simulink model "TrackShift_F1_HEV"  (R2025a)
settings: Solver=FixedStepDiscrete  StartTime=0.0  StopTime=90  FixedStep=0.25  RelTol=1e-3
model workspace (MAT data in the model file):
  TS_BRAKE = [0 0.25 0.5 0.75 1 1.25 1.5 1.75 2 2.25 2.5 2.75 ... (722 elements, 361x2)]
  TS_ENGINE_CAPACITY_L = 1.6
  TS_GAP_S = [0 0.25 0.5 0.75 1 1.25 1.5 1.75 2 2.25 2.5 2.75 ... (722 elements, 361x2)]
  TS_GRADIENT_RAD = [0 0.25 0.5 0.75 1 1.25 1.5 1.75 2 2.25 2.5 2.75 ... (722 elements, 361x2)]
  TS_HANDOVER_SOURCE = 'handover.rar / handover/export/models (production logistic models)'
  TS_SAMPLE_TIME_S = 0.25
  TS_SPEED_KPH = [0 0.25 0.5 0.75 1 1.25 1.5 1.75 2 2.25 2.5 2.75 ... (722 elements, 361x2)]
  TS_THROTTLE = [0 0.25 0.5 0.75 1 1.25 1.5 1.75 2 2.25 2.5 2.75 ... (722 elements, 361x2)]
  TS_TRACK_POS_M = [0 0.25 0.5 0.75 1 1.25 1.5 1.75 2 2.25 2.5 2.75 ... (722 elements, 361x2)]
(part 1 of 2)
settings Model: Creator=Navya  LastModifiedBy=Navya

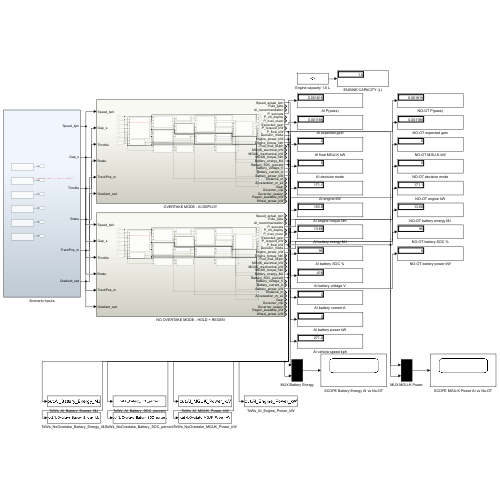
[thumbnail: Simulink's stored preview of the top-level diagram]
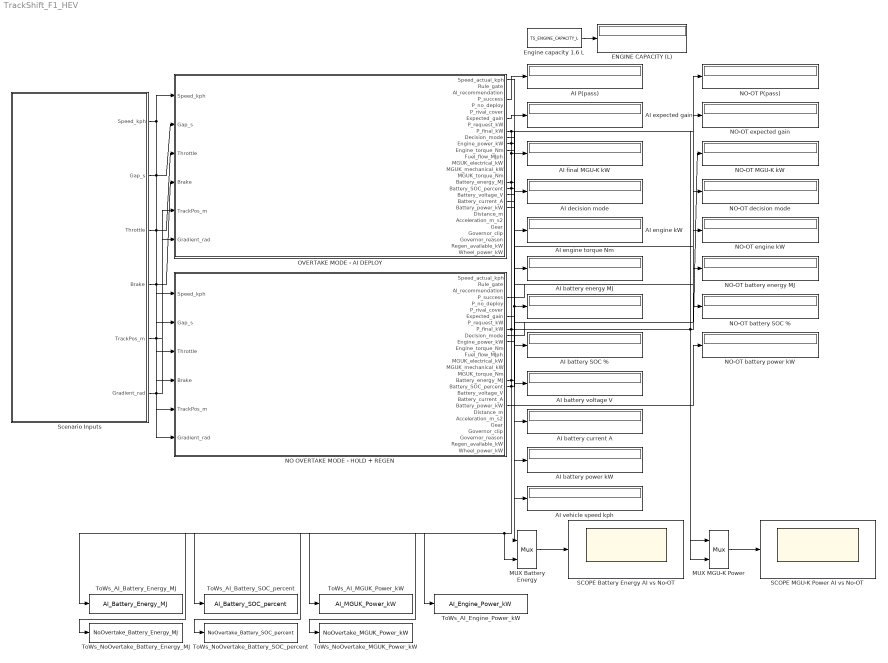
== system TrackShift_F1_HEV ==
  AI P(pass) : Display
  AI battery SOC % : Display
  AI battery current A : Display
  AI battery energy MJ : Display
  AI battery power kW : Display
  AI battery voltage V : Display
  AI decision mode : Display
  AI engine kW : Display
  AI engine torque Nm : Display
  AI expected gain : Display
  AI final MGU-K kW : Display
  AI vehicle speed kph : Display
  ENGINE CAPACITY (L) : Display
  Engine capacity 1.6 L : Constant  Value=TS_ENGINE_CAPACITY_L
  MUX Battery Energy : Mux  Inputs=2
  MUX MGU-K Power : Mux  Inputs=2
  NO OVERTAKE MODE - HOLD + REGEN : Subsystem
  NO-OT MGU-K kW : Display
  NO-OT P(pass) : Display
  NO-OT battery SOC % : Display
  NO-OT battery energy MJ : Display
  NO-OT battery power kW : Display
  NO-OT decision mode : Display
  NO-OT engine kW : Display
  NO-OT expected gain : Display
  OVERTAKE MODE - AI DEPLOY : Subsystem
  SCOPE Battery Energy AI vs No-OT : Scope
      settings: ActiveDisplayYMinimum=11.25  ActiveDisplayYMaximum=13.950000000000001
  SCOPE MGU-K Power AI vs No-OT : Scope
      settings: ActiveDisplayYMinimum=-169.375  ActiveDisplayYMaximum=324.375
  Scenario Inputs : Subsystem
  ToWs_AI_Battery_Energy_MJ : ToWorkspace  VariableName=AI_Battery_Energy_MJ  SaveFormat=Structure With Time  SampleTime=-1
  ToWs_AI_Battery_SOC_percent : ToWorkspace  VariableName=AI_Battery_SOC_percent  SaveFormat=Structure With Time  SampleTime=-1
  ToWs_AI_Engine_Power_kW : ToWorkspace  VariableName=AI_Engine_Power_kW  SaveFormat=Structure With Time  SampleTime=-1
  ToWs_AI_MGUK_Power_kW : ToWorkspace  VariableName=AI_MGUK_Power_kW  SaveFormat=Structure With Time  SampleTime=-1
  ToWs_NoOvertake_Battery_Energy_MJ : ToWorkspace  VariableName=NoOvertake_Battery_Energy_MJ  SaveFormat=Structure With Time  SampleTime=-1
  ToWs_NoOvertake_Battery_SOC_percent : ToWorkspace  VariableName=NoOvertake_Battery_SOC_percent  SaveFormat=Structure With Time  SampleTime=-1
  ToWs_NoOvertake_MGUK_Power_kW : ToWorkspace  VariableName=NoOvertake_MGUK_Power_kW  SaveFormat=Structure With Time  SampleTime=-1
  wires:
  Scenario Inputs/1(Speed_kph) -> OVERTAKE MODE - AI DEPLOY/1(Speed_kph), NO OVERTAKE MODE - HOLD + REGEN/1(Speed_kph)
  Scenario Inputs/2(Gap_s) -> OVERTAKE MODE - AI DEPLOY/2(Gap_s), NO OVERTAKE MODE - HOLD + REGEN/2(Gap_s)
  Scenario Inputs/3(Throttle) -> OVERTAKE MODE - AI DEPLOY/3(Throttle), NO OVERTAKE MODE - HOLD + REGEN/3(Throttle)
  Scenario Inputs/4(Brake) -> OVERTAKE MODE - AI DEPLOY/4(Brake), NO OVERTAKE MODE - HOLD + REGEN/4(Brake)
  Scenario Inputs/5(TrackPos_m) -> OVERTAKE MODE - AI DEPLOY/5(TrackPos_m), NO OVERTAKE MODE - HOLD + REGEN/5(TrackPos_m)
  Scenario Inputs/6(Gradient_rad) -> OVERTAKE MODE - AI DEPLOY/6(Gradient_rad), NO OVERTAKE MODE - HOLD + REGEN/6(Gradient_rad)
  Engine capacity 1.6 L/1 -> ENGINE CAPACITY (L)/1
  OVERTAKE MODE - AI DEPLOY/4(P_success) -> AI P(pass)/1
  OVERTAKE MODE - AI DEPLOY/7(Expected_gain) -> AI expected gain/1
  OVERTAKE MODE - AI DEPLOY/9(P_final_kW) -> AI final MGU-K kW/1, ToWs_AI_MGUK_Power_kW/1, MUX MGU-K Power/1
  OVERTAKE MODE - AI DEPLOY/10(Decision_mode) -> AI decision mode/1
  OVERTAKE MODE - AI DEPLOY/11(Engine_power_kW) -> AI engine kW/1, ToWs_AI_Engine_Power_kW/1
  OVERTAKE MODE - AI DEPLOY/12(Engine_torque_Nm) -> AI engine torque Nm/1
  OVERTAKE MODE - AI DEPLOY/17(Battery_energy_MJ) -> AI battery energy MJ/1, MUX Battery Energy/1, ToWs_AI_Battery_Energy_MJ/1
  OVERTAKE MODE - AI DEPLOY/18(Battery_SOC_percent) -> AI battery SOC %/1, ToWs_AI_Battery_SOC_percent/1
  OVERTAKE MODE - AI DEPLOY/19(Battery_voltage_V) -> AI battery voltage V/1
  OVERTAKE MODE - AI DEPLOY/20(Battery_current_A) -> AI battery current A/1
  OVERTAKE MODE - AI DEPLOY/21(Battery_power_kW) -> AI battery power kW/1
  OVERTAKE MODE - AI DEPLOY/1(Speed_actual_kph) -> AI vehicle speed kph/1
  NO OVERTAKE MODE - HOLD + REGEN/4(P_success) -> NO-OT P(pass)/1
  NO OVERTAKE MODE - HOLD + REGEN/7(Expected_gain) -> NO-OT expected gain/1
  NO OVERTAKE MODE - HOLD + REGEN/9(P_final_kW) -> NO-OT MGU-K kW/1, MUX MGU-K Power/2, ToWs_NoOvertake_MGUK_Power_kW/1
  NO OVERTAKE MODE - HOLD + REGEN/10(Decision_mode) -> NO-OT decision mode/1
  NO OVERTAKE MODE - HOLD + REGEN/11(Engine_power_kW) -> NO-OT engine kW/1
  NO OVERTAKE MODE - HOLD + REGEN/17(Battery_energy_MJ) -> MUX Battery Energy/2, ToWs_NoOvertake_Battery_Energy_MJ/1, NO-OT battery energy MJ/1
  NO OVERTAKE MODE - HOLD + REGEN/18(Battery_SOC_percent) -> NO-OT battery SOC %/1, ToWs_NoOvertake_Battery_SOC_percent/1
  NO OVERTAKE MODE - HOLD + REGEN/21(Battery_power_kW) -> NO-OT battery power kW/1
  MUX Battery Energy/1 -> SCOPE Battery Energy AI vs No-OT/1
  MUX MGU-K Power/1 -> SCOPE MGU-K Power AI vs No-OT/1
